simulink model "L1OF2_SecondOrder_M2_2_FRNEU"  (Simulink 7.8)
settings: Solver=ode45  StartTime=0.0  StopTime=10.0  FixedStep=1e-4
values from neighbouring files (symbols this model uses):
  a2 = M.den{1}(1)    [L1OF2SecondOrder2_2.m]
  Am = A_Db'    [L1OF2SecondOrder2_2.m]    (also in MaximiereL1NG.m)
  bm = c_Db'    [L1OF2SecondOrder2_2.m]    (also in MaximiereL1NG.m)
  cm = b_Db'    [L1OF2SecondOrder2_2.m]    (also in MaximiereL1NG.m)
  epsilon = 1.3    [L1OF2SecondOrder2_2.m]
  Gain = -Phi\mu1    [L1OF2SecondOrder2_2.m]
  ICy = 0    [L1OF2SecondOrder2_2.m]
  KmY = 2.4    [L1OF2SecondOrder2_2.m]
  kvy = 0    [L1OF2SecondOrder2_2.m]
  m = 19    [L1OF2SecondOrder2_2.m]
  M = 1/(7.713778844*s^2+10.06175892*s+1)    [L1OF2SecondOrder2_2.m]    (also in MaximiereL1NG.m = 1/(1.566434557*s^2+3.001699185*s+1))
  pD = p(2)-a1/a2    [L1OF2SecondOrder2_2.m]
  pI = p(4)    [L1OF2SecondOrder2_2.m]
  pK = p(3)-a0/a2    [L1OF2SecondOrder2_2.m]
  Ref_Amplitude = 0.3/Ref_Frequenz^2    (= 0.0697804295057)    [L1OF2SecondOrder2_2.m]
  Ref_Frequenz = 2*pi*0.33    (= 2.07345115137)    [L1OF2SecondOrder2_2.m]
  ST = 0.0005    [L1OF2SecondOrder2_2.m]
  Tt = 0.0667    [L1OF2SecondOrder2_2.m]
undefined symbols (not defined in the file or in its folder): d1, d2, delta, FpxLookUp1, FpxLookUp2, FpyLookUp1, FpyLookUp2, ICphi, ICvphi, ICvx, ICvy, ICx, J, KmX, kvphi, kvx, KX1, KX2, KY1, KY2, Ox1, Ox2, Oy1, Oy2, phx, phy, sigma, Tk, Vx1, Vx2, Vy1, Vy2, xLookUp1, xLookUp2, yLookUp1, yLookUp2
libraries: cstblocks x3, simulink x3
settings Model: Creator=Markus  LastModifiedBy=Markus

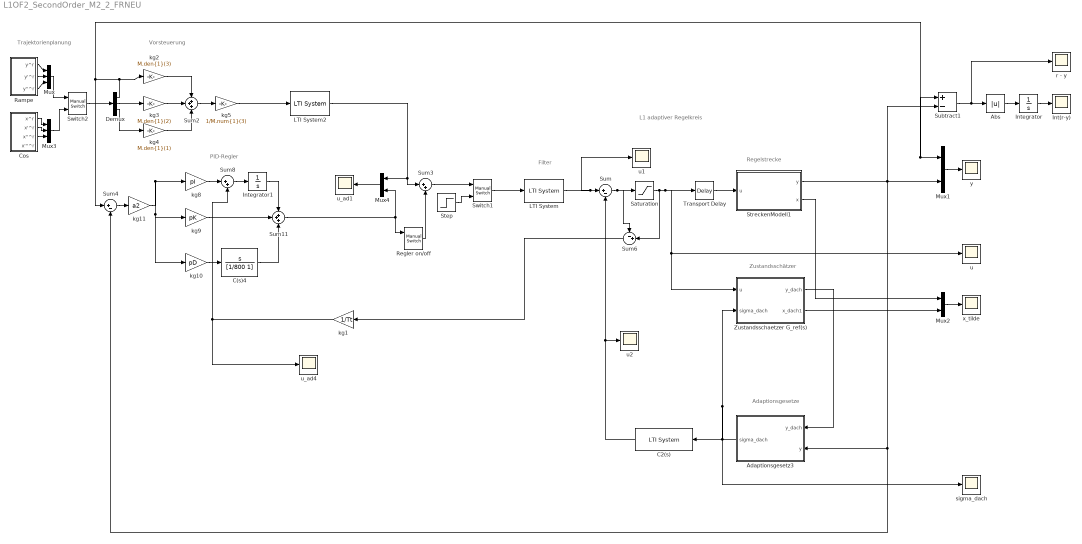
== system L1OF2_SecondOrder_M2_2_FRNEU ==
  note: Filter
  note: Zustandsschätzer
  note: Adaptionsgesetze
  note: Regelstrecke
  note: Trajektorienplanung
  note: Vorsteuerung
  note: L1 adaptiver Regelkreis
  note: PID-Regler
  Abs : Abs
  Adaptionsgesetz3 : Subsystem
  C(s)4 : TransferFcn  Numerator=[1 0]  Denominator=[1/800 1]
  C2(s) : cstblocks/LTI System  sys=C2  IC=[]
  Cos : Subsystem
  Demux : Demux  Outputs=3
  Int(r-y) : Scope
      settings: TimeRange=6  YMin=0.18335  YMax=0.18445  SaveName=ScopeData2
  Integrator : Integrator
  Integrator1 : Integrator
  LTI System : cstblocks/LTI System  sys=C  IC=[]
  LTI System2 : cstblocks/LTI System  sys=C_inv  IC=[]
  Mux : Mux  Inputs=3
  Mux1 : Mux  Inputs=2
  Mux2 : Mux  Inputs=2
  Mux3 : Mux  Inputs=3
  Mux4 : Mux  Inputs=3
  Rampe : Subsystem
  Regler on/off : simulink/Signal Routing/Manual Switch  sw=1  action=0  varsize=off
  Saturation : Saturate  UpperLimit=3  LowerLimit=-3
  Step : Step  After=0.06  SampleTime=0
  StreckenModell1 : Subsystem
  Subtract1 : Sum  Inputs=+-
  Sum : Sum  Inputs=|+-
  Sum11 : Sum  Inputs=+++
  Sum2 : Sum  Inputs=+++
  Sum3 : Sum  Inputs=|++
  Sum4 : Sum  Inputs=|+-
  Sum6 : Sum  Inputs=-+|
  Sum8 : Sum  Inputs=|++
  Switch1 : simulink/Signal Routing/Manual Switch  sw=1  action=0  varsize=off
  Switch2 : simulink/Signal Routing/Manual Switch  sw=1  action=0  varsize=off
  Transport Delay : TransportDelay  DelayTime=0.000
  Zustandsschaetzer G_ref(s) : Subsystem
  kg1 : Gain  Gain=1/Tt
  kg10 : Gain  Gain=pD
  kg11 : Gain  Gain=a2
  kg2 : Gain  Gain=M.den{1}(3)
  kg3 : Gain  Gain=M.den{1}(2)
  kg4 : Gain  Gain=M.den{1}(1)
  kg5 : Gain  Gain=1/M.num{1}(3)
  kg8 : Gain  Gain=pI
  kg9 : Gain  Gain=pK
  r - y : Scope
      settings: TimeRange=10  YMin=6e-012  YMax=2.6e-011  SaveName=simoutE
  sigma_dach : Scope
      settings: TimeRange=10  YMin=-0.04  YMax=0.075  SaveName=simoutS
  u : Scope
      settings: TimeRange=8  YMin=-2  YMax=2  SaveName=simoutU
  u1 : Scope
      settings: TimeRange=10  YMin=0.37  YMax=0.56  SaveName=ScopeData13
  u2 : Scope
      settings: TimeRange=10  YMin=-17.5  YMax=37.5  SaveName=ScopeData12
  u_ad1 : Scope
      settings: TimeRange=20  YMin=-50  YMax=110  SaveName=simoutV
  u_ad4 : Scope
      settings: TimeRange=20  YMin=-170  YMax=50  SaveName=simoutV1
  x_tilde : Scope
      settings: TimeRange=10  YMin=-0.0075  YMax=0.0475  SaveName=simoutU1
  y : Scope
      settings: TimeRange=4  YMin=0.07778  YMax=0.07781  SaveName=simout
  wires:
  Mux1/1 -> y/1
  Adaptionsgesetz3/1(sigma_dach) -> Zustandsschaetzer G_ref(s)/2(sigma_dach), sigma_dach/1, C2(s)/1
  Zustandsschaetzer G_ref(s)/1(y_dach) -> Adaptionsgesetz3/1(y_dach)
  LTI System/1 -> Sum/1, u1/1
  C2(s)/1 -> Sum/2, u2/1
  Subtract1/1 -> r - y/1, Abs/1
  Integrator/1 -> Int(r-y)/1
  Abs/1 -> Integrator/1
  Sum/1 -> Saturation/1, Sum6/1
  Saturation/1 -> Zustandsschaetzer G_ref(s)/1(u), u/1, Transport Delay/1, Sum6/2
  Switch1/1 -> LTI System/1
  StreckenModell1/1(y) -> Mux1/2, Adaptionsgesetz3/2(y), Sum4/2, Subtract1/2
  Transport Delay/1 -> StreckenModell1/1(u)
  Mux2/1 -> x_tilde/1
  StreckenModell1/2(x) -> Mux2/1
  Zustandsschaetzer G_ref(s)/2(x_dach1) -> Mux2/2
  Demux/1 -> kg2/1, Sum4/1, Subtract1/1, Mux1/1
  Demux/2 -> kg3/1
  Demux/3 -> kg4/1
  kg3/1 -> Sum2/2
  kg4/1 -> Sum2/3
  Sum2/1 -> kg5/1
  kg2/1 -> Sum2/1
  Rampe/1(y^r) -> Mux/1
  Rampe/2(y'^r) -> Mux/2
  Rampe/3(y''^r) -> Mux/3
  Mux/1 -> Switch2/1
  Switch2/1 -> Demux/1
  Mux3/1 -> Switch2/2
  Cos/1(x^r) -> Mux3/1
  Cos/2(x'^r) -> Mux3/2
  Cos/3(x''^r) -> Mux3/3
  Mux4/1 -> u_ad1/1
  Regler on/off/1 -> Sum3/2
  Sum3/1 -> Switch1/1
  kg5/1 -> LTI System2/1
  LTI System2/1 -> Sum3/1, Mux4/1
  kg1/1 -> Sum8/2, u_ad4/1
  Integrator1/1 -> Sum11/1
  kg9/1 -> Sum11/2
  kg8/1 -> Sum8/1
  Sum8/1 -> Integrator1/1
  kg10/1 -> C(s)4/1
  C(s)4/1 -> Sum11/3
  kg11/1 -> kg8/1, kg9/1, kg10/1
  Step/1 -> Switch1/2
  Sum4/1 -> kg11/1
  Sum11/1 -> Regler on/off/1, Mux4/3
  Sum6/1 -> kg1/1

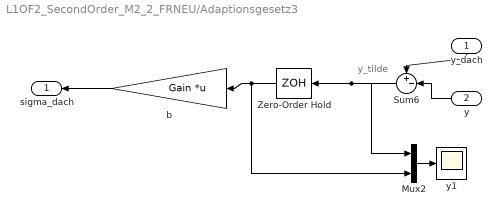
== system L1OF2_SecondOrder_M2_2_FRNEU/Adaptionsgesetz3 ==
  note: y_tilde
  y_dach : Inport
  y : Inport  Port=2
  Mux2 : Mux  Inputs=2
  Sum6 : Sum  Inputs=+-|
  Zero-Order Hold : ZeroOrderHold  SampleTime=ST
  b : Gain  Gain=Gain  Multiplication=Matrix(K*u)
  y1 : Scope
      settings: TimeRange=10  YMin=-0.004500000000000001  YMax=0  SaveName=ScopeData4
  sigma_dach : Outport
  wires:
  Sum6/1 -> Zero-Order Hold/1, Mux2/1
  y_dach/1 -> Sum6/1
  y/1 -> Sum6/2
  Zero-Order Hold/1 -> b/1, Mux2/2
  b/1 -> sigma_dach/1
  Mux2/1 -> y1/1

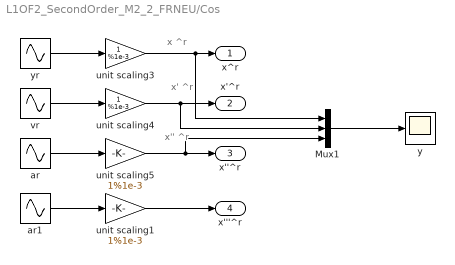
== system L1OF2_SecondOrder_M2_2_FRNEU/Cos ==
  note: x ^r
  note: x' ^r
  note: x'' ^r
  Mux1 : Mux  Inputs=3
  ar : Sin  Amplitude=-Ref_Amplitude*Ref_Frequenz^2  Frequency=Ref_Frequenz  Phase=pi/2  SampleTime=0
  ar1 : Sin  Amplitude=Ref_Amplitude*Ref_Frequenz^3  Frequency=Ref_Frequenz  SampleTime=0
  unit scaling1 : Gain  Gain=1%1e-3
  unit scaling3 : Gain  Gain=1 %1e-3
  unit scaling4 : Gain  Gain=1 %1e-3
  unit scaling5 : Gain  Gain=1%1e-3
  vr : Sin  Amplitude=-Ref_Amplitude*Ref_Frequenz  Frequency=Ref_Frequenz  SampleTime=0
  y : Scope
      settings: TimeRange=20  YMin=-0.3  YMax=0.25  SaveName=simout1
  yr : Sin  Amplitude=Ref_Amplitude  Frequency=Ref_Frequenz  Phase=pi/2  SampleTime=0
  x^r : Outport
  x'^r : Outport  Port=2
  x''^r : Outport  Port=3
  x'''^r : Outport  Port=4
  wires:
  ar/1 -> unit scaling5/1
  vr/1 -> unit scaling4/1
  yr/1 -> unit scaling3/1
  unit scaling3/1 -> x^r/1, Mux1/1
  unit scaling4/1 -> x'^r/1, Mux1/2
  unit scaling5/1 -> x''^r/1, Mux1/3
  Mux1/1 -> y/1
  ar1/1 -> unit scaling1/1
  unit scaling1/1 -> x'''^r/1

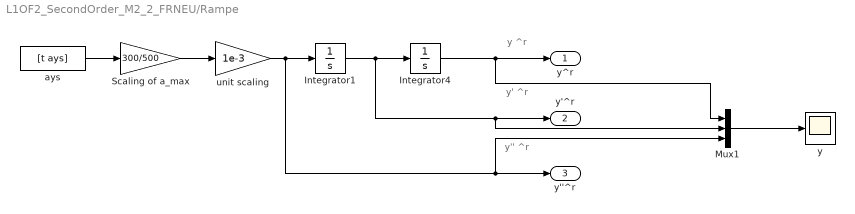
== system L1OF2_SecondOrder_M2_2_FRNEU/Rampe ==
  note: y ^r
  note: y' ^r
  note: y'' ^r
  Integrator1 : Integrator  InitialCondition=ICvy
  Integrator4 : Integrator  InitialCondition=ICy
  Mux1 : Mux  Inputs=3
  Scaling of a_max : Gain  Gain=300/500
  ays : FromWorkspace  VariableName=[t ays]  SampleTime=0
  unit scaling : Gain  Gain=1e-3
  y : Scope
      settings: TimeRange=20  YMin=-0.005  YMax=0.08  SaveName=simout2
  y^r : Outport
  y'^r : Outport  Port=2
  y''^r : Outport  Port=3
  wires:
  ays/1 -> Scaling of a_max/1
  Scaling of a_max/1 -> unit scaling/1
  Integrator1/1 -> Integrator4/1, y'^r/1, Mux1/2
  unit scaling/1 -> Integrator1/1, y''^r/1, Mux1/3
  Integrator4/1 -> y^r/1, Mux1/1
  Mux1/1 -> y/1

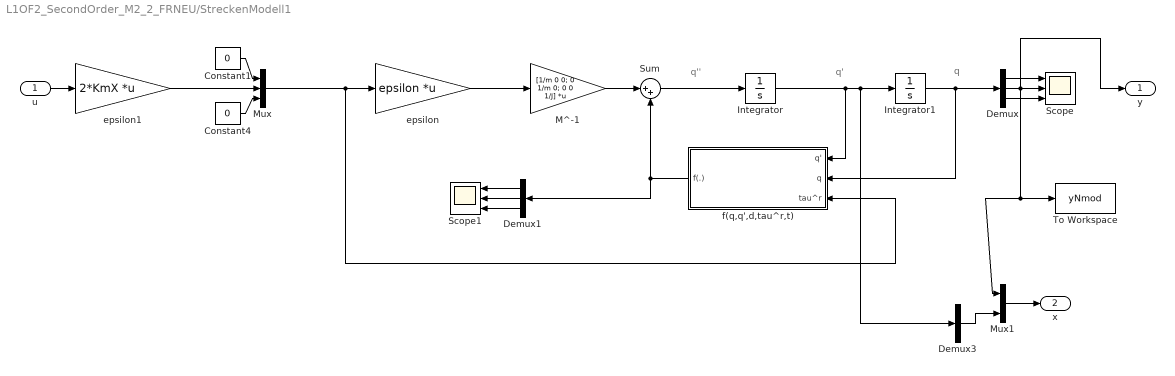
== system L1OF2_SecondOrder_M2_2_FRNEU/StreckenModell1 ==
  note: q
  note: q'
  note: q''
  u : Inport
  Constant1 : Constant  Value=0
  Constant4 : Constant  Value=0
  Demux : Demux  Outputs=3
  Demux1 : Demux  Outputs=3
  Demux3 : Demux  Outputs=3
  Integrator : Integrator  InitialCondition=[ICvx;ICvy;ICvphi]
  Integrator1 : Integrator  InitialCondition=[ICx;ICy;ICphi]
  M^-1 : Gain  Gain=[1/m 0 0; 0 1/m 0; 0 0 1/J]  Multiplication=Matrix(K*u)
  Mux : Mux  Inputs=3
  Mux1 : Mux  Inputs=2
  Scope : Scope  NumInputPorts=3
      settings: YMin=0.0014~0.0425~-1.73472e-018  YMax=0.0029~0.0625~0.08
  Scope1 : Scope  NumInputPorts=3
      settings: YMin=-1~1.1~-1  YMax=1~2.6~1  SaveName=ScopeData2
  Sum : Sum  Inputs=|++
  To Workspace : ToWorkspace  VariableName=yNmod  SampleTime=-1  SaveFormat=Structure With Time
  epsilon : Gain  Gain=epsilon  Multiplication=Matrix(K*u)
  epsilon1 : Gain  Gain=2*KmX  Multiplication=Matrix(K*u)
  f(q,q',d,tau^r,t) : Subsystem
  y : Outport
  x : Outport  Port=2
  wires:
  Demux3/2 -> Mux1/2
  Mux1/1 -> x/1
  Constant4/1 -> Mux/3
  Constant1/1 -> Mux/1
  Mux/1 -> f(q,q',d,tau^r,t)/3(tau^r), epsilon/1
  Demux1/3 -> Scope1/3
  Demux1/2 -> Scope1/2
  Demux1/1 -> Scope1/1
  f(q,q',d,tau^r,t)/1(f(.)) -> Demux1/1, Sum/2
  epsilon/1 -> M^-1/1
  Integrator1/1 -> f(q,q',d,tau^r,t)/2(q), Demux/1
  Sum/1 -> Integrator/1
  M^-1/1 -> Sum/1
  Integrator/1 -> Demux3/1, Integrator1/1, f(q,q',d,tau^r,t)/1(q')
  Demux/3 -> Scope/3
  Demux/2 -> Mux1/1, To Workspace/1, y/1, Scope/2
  Demux/1 -> Scope/1
  u/1 -> epsilon1/1
  epsilon1/1 -> Mux/2

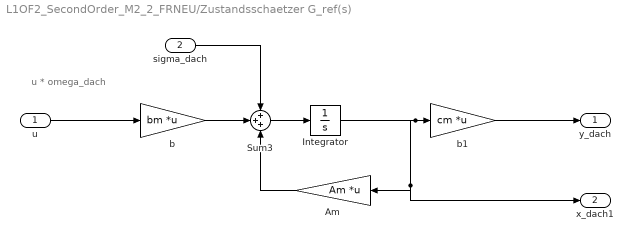
== system L1OF2_SecondOrder_M2_2_FRNEU/Zustandsschaetzer G_ref(s) ==
  note: u * omega_dach
  u : Inport
  sigma_dach : Inport  Port=2
  Am : Gain  Gain=Am  Multiplication=Matrix(K*u)
  Integrator : Integrator
  Sum3 : Sum  Inputs=+++
  b : Gain  Gain=bm  Multiplication=Matrix(K*u)
  b1 : Gain  Gain=cm  Multiplication=Matrix(K*u)
  y_dach : Outport
  x_dach1 : Outport  Port=2
  wires:
  Integrator/1 -> b1/1, Am/1, x_dach1/1
  Sum3/1 -> Integrator/1
  Am/1 -> Sum3/3
  b/1 -> Sum3/2
  sigma_dach/1 -> Sum3/1
  b1/1 -> y_dach/1
  u/1 -> b/1

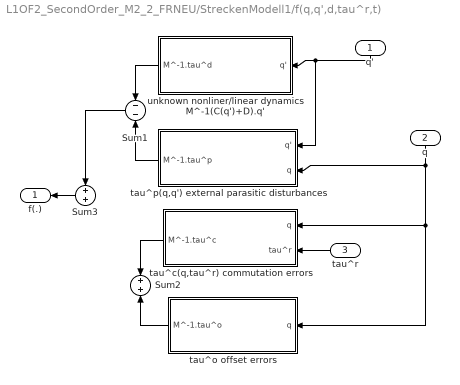
== system L1OF2_SecondOrder_M2_2_FRNEU/StreckenModell1/f(q,q',d,tau^r,t) ==
  q' : Inport
  q : Inport  Port=2
  tau^r : Inport  Port=3
  Sum1 : Sum  Inputs=--
  Sum2 : Sum
  Sum3 : Sum
  tau^c(q,tau^r) commutation errors : Subsystem
  tau^o offset errors : Subsystem
  tau^p(q,q') external parasitic disturbances : Subsystem
  unknown nonliner/linear dynamics M^-1(C(q')+D).q' : Subsystem
  f(.) : Outport
  wires:
  Sum3/1 -> f(.)/1
  tau^r/1 -> tau^c(q,tau^r) commutation errors/2(tau^r)
  q/1 -> tau^o offset errors/1(q), tau^c(q,tau^r) commutation errors/1(q), tau^p(q,q') external parasitic disturbances/2(q)
  q'/1 -> unknown nonliner/linear dynamics M^-1(C(q')+D).q'/1(q'), tau^p(q,q') external parasitic disturbances/1(q')
  Sum1/1 -> Sum3/1
  unknown nonliner/linear dynamics M^-1(C(q')+D).q'/1(M^-1.tau^d) -> Sum1/1
  tau^c(q,tau^r) commutation errors/1(M^-1.tau^c) -> Sum2/1
  tau^p(q,q') external parasitic disturbances/1(M^-1.tau^p) -> Sum1/2
  tau^o offset errors/1(M^-1.tau^o) -> Sum2/2

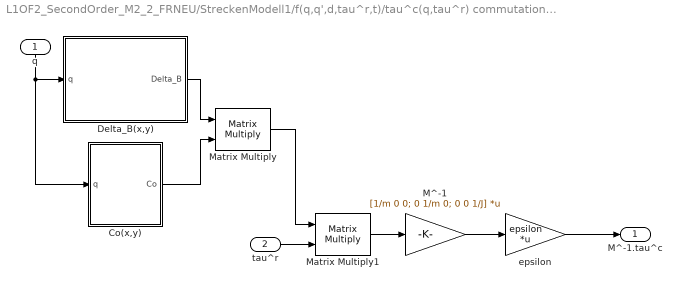
== system L1OF2_SecondOrder_M2_2_FRNEU/StreckenModell1/f(q,q',d,tau^r,t)/tau^c(q,tau^r) commutation errors ==
  q : Inport
  tau^r : Inport  Port=2
  Co(x,y) : MATLAB Function  TreatAsAtomicUnit=on
  Delta_B(x,y) : MATLAB Function  TreatAsAtomicUnit=on
  "M^-1  " : Gain  Gain=[1/m 0 0; 0 1/m 0; 0 0 1/J]  Multiplication=Matrix(K*u)
  Matrix Multiply : Product  Multiplication=Matrix(*)
  Matrix Multiply1 : Product  Multiplication=Matrix(*)
  epsilon : Gain  Gain=epsilon  Multiplication=Matrix(K*u)
  M^-1.tau^c : Outport
  wires:
  "M^-1  "/1 -> epsilon/1
  epsilon/1 -> M^-1.tau^c/1
  tau^r/1 -> Matrix Multiply1/2
  q/1 -> Co(x,y)/1(q), Delta_B(x,y)/1(q)
  Matrix Multiply1/1 -> "M^-1  "/1
  Matrix Multiply/1 -> Matrix Multiply1/1
  Co(x,y)/1(Co) -> Matrix Multiply/2
  Delta_B(x,y)/1(Delta_B) -> Matrix Multiply/1

== system L1OF2_SecondOrder_M2_2_FRNEU/StreckenModell1/f(q,q',d,tau^r,t)/tau^o offset errors ==
  q : Inport
  Delta_B(x,y) : MATLAB Function  TreatAsAtomicUnit=on
  "M^-1  " : Gain  Gain=[1/m 0 0; 0 1/m 0; 0 0 1/J]  Multiplication=Matrix(K*u)
  Matrix Multiply1 : Product  Multiplication=Matrix(*)
  sigma : Constant  Value=sigma
  M^-1.tau^o : Outport
  wires:
  sigma/1 -> Matrix Multiply1/2
  Matrix Multiply1/1 -> "M^-1  "/1
  "M^-1  "/1 -> M^-1.tau^o/1
  q/1 -> Delta_B(x,y)/1(q)
  Delta_B(x,y)/1(Bp) -> Matrix Multiply1/1

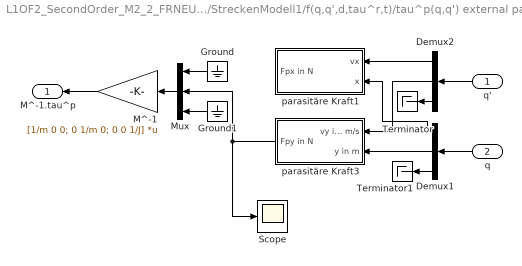
== system L1OF2_SecondOrder_M2_2_FRNEU/StreckenModell1/f(q,q',d,tau^r,t)/tau^p(q,q') external parasitic disturbances ==
  q' : Inport
  q : Inport  Port=2
  Demux1 : Demux  Outputs=3
  Demux2 : Demux  Outputs=3
  Ground : Ground
  Ground1 : Ground
  "M^-1  " : Gain  Gain=[1/m 0 0; 0 1/m 0; 0 0 1/J]  Multiplication=Matrix(K*u)
  Mux : Mux  Inputs=3
  Scope : Scope
      settings: YMin=-4.06576e-020  YMax=0.0007  SaveName=ScopeData19
  Terminator : Terminator
  Terminator1 : Terminator
  parasitäre Kraft1 : Subsystem
  parasitäre Kraft3 : Subsystem
  M^-1.tau^p : Outport
  wires:
  Ground1/1 -> Mux/3
  "M^-1  "/1 -> M^-1.tau^p/1
  Mux/1 -> "M^-1  "/1
  q/1 -> Demux1/1
  q'/1 -> Demux2/1
  parasitäre Kraft3/1(Fpy in N) -> Scope/1, Mux/2
  Demux2/2 -> parasitäre Kraft3/1(vy in m/s)
  Demux1/3 -> Terminator1/1
  Demux2/3 -> Terminator/1
  Demux2/1 -> parasitäre Kraft1/1(vx)
  Demux1/2 -> parasitäre Kraft3/2(y in m)
  Demux1/1 -> parasitäre Kraft1/2(x)
  Ground/1 -> Mux/1

== system L1OF2_SecondOrder_M2_2_FRNEU/StreckenModell1/f(q,q',d,tau^r,t)/unknown nonliner/linear dynamics M^-1(C(q')+D).q' ==
  q' : Inport
  C(q').q' : Subsystem
  "M^-1 " : Gain  Gain=[1/m 0 0; 0 1/m 0; 0 0 1/J]  Multiplication=Matrix(K*u)
  M^-1.D : Gain  Gain=[kvx/m 0 0; 0 kvy/m 0; 0 0 kvphi/J]  Multiplication=Matrix(K*u)
  Sum1 : Sum
  M^-1.tau^d : Outport
  wires:
  M^-1.D/1 -> Sum1/1
  Sum1/1 -> M^-1.tau^d/1
  "M^-1 "/1 -> Sum1/2
  q'/1 -> C(q').q'/1(q'), M^-1.D/1
  C(q').q'/1(C(q').q') -> "M^-1 "/1

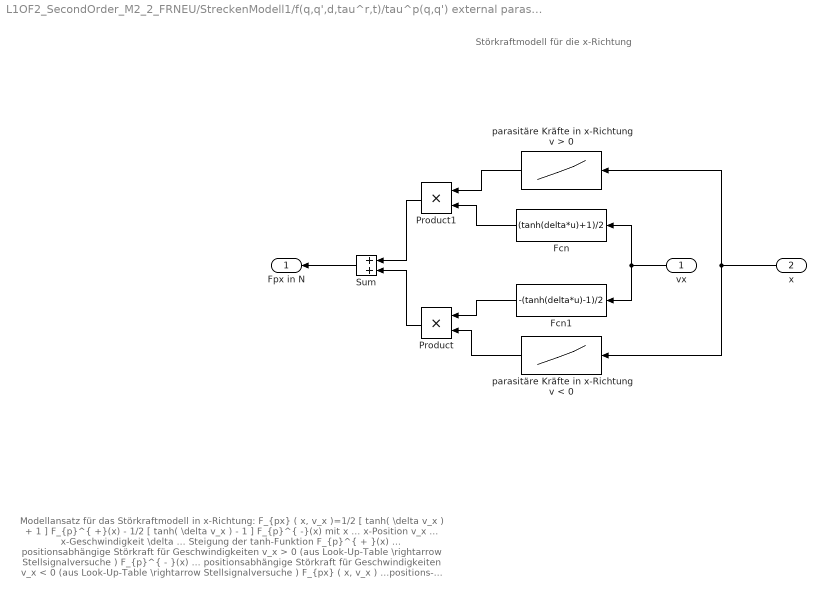
== system L1OF2_SecondOrder_M2_2_FRNEU/StreckenModell1/f(q,q',d,tau^r,t)/tau^p(q,q') external parasitic disturbances/parasitäre Kraft1 ==
  note: Modellansatz für das Störkraftmodell in x-Richtung:
      |
      | F_{px} ( x, v_x )=1/2 [ tanh(  \delta  v_x ) + 1 ] F_{p}^{  +}(x)  -  1/2 [ tanh( \delta  v_x )  - 1 ]  F_{p}^{  -}(x)
      |
      | mit
      |
      | x    ... x-Position
      | v_x  ... x-Geschwindigkeit
      | \delta   ... Steigung der tanh-Funktion
      |
      | F_{p}^{  + }(x)          ... positionsabhängige Störkraft für Geschwindigkeiten v_x   >  0  (aus Look-Up-Table \rightarrow Stellsignalversuche )
      | F_{p}^{  - }(x)           ... positionsabhängige Störkraft für Geschwindigkeiten v_x   <  0  (aus Look-Up-Table \rightarrow Stellsignalversuche )
      | F_{px} ( x, v_x ) ...positions- und richtungsabhängige Störkraft
  note: Störkraftmodell für die x-Richtung
  vx : Inport
  x : Inport  Port=2
  Fcn : Fcn  Expr=(tanh(delta*u)+1)/2
  Fcn1 : Fcn  Expr=-(tanh(delta*u)-1)/2
  Product : Product  RndMeth=Zero
  Product1 : Product  RndMeth=Zero
  Sum : Sum
  parasitäre Kräfte in x-Richtung v < 0 : Lookup_n-D  NumberOfTableDimensions=1  BreakpointsForDimension1=fliplr(xLookUp2')*1e-3+Vx2  Table=fliplr(FpxLookUp2')*KX2+Ox2  InterpMethod=Cubic spline  RndMeth=Simplest  InputSameDT=on
  parasitäre Kräfte in x-Richtung v > 0 : Lookup_n-D  NumberOfTableDimensions=1  BreakpointsForDimension1=xLookUp1*1e-3+Vx1  Table=FpxLookUp1*KX1+Ox1  InterpMethod=Cubic spline  RndMeth=Simplest  InputSameDT=on
  Fpx in N : Outport
  wires:
  vx/1 -> Fcn1/1, Fcn/1
  Sum/1 -> Fpx in N/1
  Product/1 -> Sum/2
  Product1/1 -> Sum/1
  Fcn/1 -> Product1/2
  parasitäre Kräfte in x-Richtung v > 0/1 -> Product1/1
  Fcn1/1 -> Product/1
  parasitäre Kräfte in x-Richtung v < 0/1 -> Product/2
  x/1 -> parasitäre Kräfte in x-Richtung v < 0/1, parasitäre Kräfte in x-Richtung v > 0/1

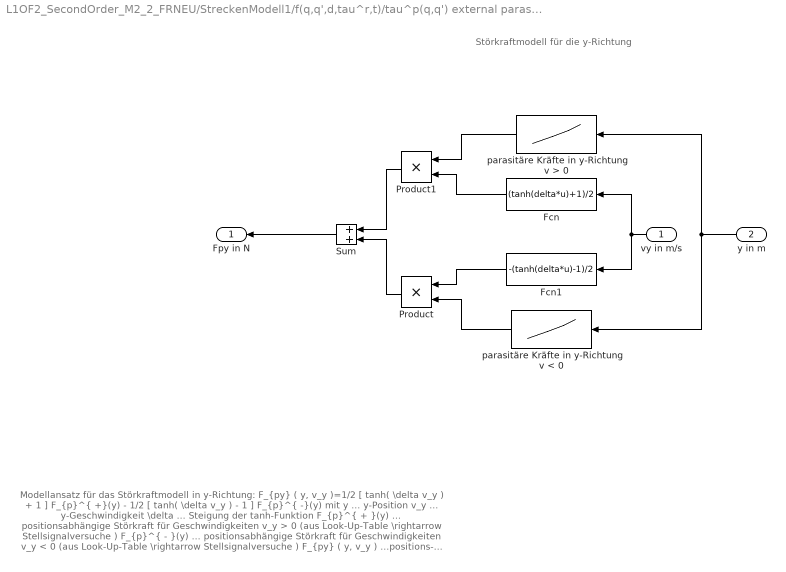
== system L1OF2_SecondOrder_M2_2_FRNEU/StreckenModell1/f(q,q',d,tau^r,t)/tau^p(q,q') external parasitic disturbances/parasitäre Kraft3 ==
  note: Störkraftmodell für die y-Richtung
  note: Modellansatz für das Störkraftmodell in y-Richtung:
      |
      | F_{py} ( y, v_y )=1/2 [ tanh(  \delta  v_y ) + 1 ] F_{p}^{  +}(y)  -  1/2 [ tanh( \delta  v_y )  - 1 ]  F_{p}^{  -}(y)
      |
      | mit
      |
      | y    ... y-Position
      | v_y  ... y-Geschwindigkeit
      | \delta   ... Steigung der tanh-Funktion
      |
      | F_{p}^{  + }(y)          ... positionsabhängige Störkraft für Geschwindigkeiten v_y   >  0  (aus Look-Up-Table \rightarrow Stellsignalversuche )
      | F_{p}^{  - }(y)           ... positionsabhängige Störkraft für Geschwindigkeiten v_y   <  0  (aus Look-Up-Table \rightarrow Stellsignalversuche )
      | F_{py} ( y, v_y ) ...positions- und richtungsabhängige Störkraft
  vy in m/s : Inport
  y in m : Inport  Port=2
  Fcn : Fcn  Expr=(tanh(delta*u)+1)/2
  Fcn1 : Fcn  Expr=-(tanh(delta*u)-1)/2
  Product : Product  RndMeth=Zero
  Product1 : Product  RndMeth=Zero
  Sum : Sum
  parasitäre Kräfte in y-Richtung v < 0 : Lookup_n-D  NumberOfTableDimensions=1  BreakpointsForDimension1=fliplr(yLookUp2')*1e-3+Vy2  Table=fliplr(FpyLookUp2')*KY2+Oy2  InterpMethod=Cubic spline  RndMeth=Simplest  InputSameDT=on
  parasitäre Kräfte in y-Richtung v > 0 : Lookup_n-D  NumberOfTableDimensions=1  BreakpointsForDimension1=yLookUp1*1e-3+Vy1  Table=FpyLookUp1*KY1+Oy1  InterpMethod=Cubic spline  RndMeth=Simplest  InputSameDT=on
  Fpy in N : Outport
  wires:
  parasitäre Kräfte in y-Richtung v < 0/1 -> Product/2
  parasitäre Kräfte in y-Richtung v > 0/1 -> Product1/1
  Product/1 -> Sum/2
  Product1/1 -> Sum/1
  Fcn/1 -> Product1/2
  Fcn1/1 -> Product/1
  Sum/1 -> Fpy in N/1
  vy in m/s/1 -> Fcn/1, Fcn1/1
  y in m/1 -> parasitäre Kräfte in y-Richtung v > 0/1, parasitäre Kräfte in y-Richtung v < 0/1

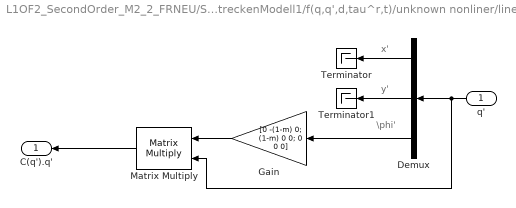
== system L1OF2_SecondOrder_M2_2_FRNEU/StreckenModell1/f(q,q',d,tau^r,t)/unknown nonliner/linear dynamics M^-1(C(q')+D).q'/C(q').q' ==
  note: \phi'
  note: y'
  note: x'
  q' : Inport
  Demux : Demux  Outputs=3
  Gain : Gain  Gain=[0 -(1-m) 0; (1-m) 0 0; 0 0 0]
  Matrix Multiply : Product  Multiplication=Matrix(*)
  Terminator : Terminator
  Terminator1 : Terminator
  C(q').q' : Outport
  wires:
  Demux/3 -> Gain/1
  Matrix Multiply/1 -> C(q').q'/1
  Gain/1 -> Matrix Multiply/1
  Demux/2 -> Terminator1/1
  Demux/1 -> Terminator/1
  q'/1 -> Matrix Multiply/2, Demux/1

== matlab function StreckenModell1/f(q,q',d,tau^r,t)/tau^c(q,tau^r) commutation errors/Co(x,y) ==
  data: q input double; Co output double; Tk parameter double; KmX parameter double; KmY parameter double; phx parameter double; phy parameter double; d1 parameter double; d2 parameter double
function Co = compute_Co(q,Tk,KmX,KmY,phx,phy,d1,d2)
%#codegen
x=q(1);
y=q(2);

% Flussdichte entlang der x- und y-Richtungen
B1x=sin(2*pi/Tk*x+phx+pi/2); %+
B2x=cos(2*pi/Tk*x+phx-pi/2); %-
B1y=sin(2*pi/Tk*y+phy);
B2y=cos(2*pi/Tk*y+phy);


Co =[B1x/(2*KmX)    0         d1*KmX*B1x/(2*(d1^2*KmX^2+d2^2*KmY^2));
     B2x/(2*KmX)    0         d1*KmX*B2x/(2*(d1^2*KmX^2+d2^2*KmY^2));
     B1x/(2*KmX)    0        -d1*KmX*B1x/(2*(d1^2*KmX^2+d2^2*KmY^2));
     B2x/(2*KmX)    0        -d1*KmX*B2x/(2*(d1^2*KmX^2+d2^2*KmY^2));
        0        B1y/(2*KmY) -d2*KmY*B1y/(2*(d1^2*KmX^2+d2^2*KmY^2));
        0        B2y/(2*KmY) -d2*KmY*B2y/(2*(d1^2*KmX^2+d2^2*KmY^2));
        0        B1y/(2*KmY)  d2*KmY*B1y/(2*(d1^2*KmX^2+d2^2*KmY^2));
        0        B2y/(2*KmY)  d2*KmY*B2y/(2*(d1^2*KmX^2+d2^2*KmY^2))];

== matlab function StreckenModell1/f(q,q',d,tau^r,t)/tau^c(q,tau^r) commutation errors/Delta_B(x,y) ==
  data: q input double; Delta_B output double; Tk parameter double; KmX parameter double; KmY parameter double; phx parameter double; phy parameter double; d1 parameter double; d2 parameter double
function Delta_B = compute_Delta_B(q,Tk,KmX,KmY,phx,phy,d1,d2)
%#codegen
x=q(1);
y=q(2);

% Flussdichte entlang der x- und y-Richtungen
B1x=KmX*sin(2*pi/Tk*x+phx+pi/2); %+
B2x=KmX*cos(2*pi/Tk*x+phx-pi/2); %-
B1y=KmY*sin(2*pi/Tk*y+phy);
B2y=KmY*cos(2*pi/Tk*y+phy);

% nominelles Feld
B =[   B1x    B2x     B1x     B2x      0       0      0      0;
        0      0       0       0      B1y     B2y    B1y    B2y;
     d1*B1x d1*B2x -d1*B1x -d1*B2x -d2*B1y -d2*B2y d2*B1y d2*B2y];

 
% Fehlerhaftes Magnetfeld
maxBp=0.4704;
B1xp=0.4851*tanh(0.1877*sinh(3.104*B1x))/maxBp; 
B2xp=0.4851*tanh(0.1877*sinh(3.104*B2x))/maxBp; 
B1yp=0.4851*tanh(0.1877*sinh(3.104*B1y))/maxBp; 
B2yp=0.4851*tanh(0.1877*sinh(3.104*B2y))/maxBp; 

Bp =[   B1xp    B2xp    B1xp     B2xp      0       0       0       0;
         0       0       0        0       B1yp    B2yp    B1yp    B2yp;
     d1*B1xp d1*B2xp -d1*B1xp -d1*B2xp -d2*B1yp -d2*B2yp d2*B1yp d2*B2yp];
 
Delta_B=Bp-B;

== matlab function StreckenModell1/f(q,q',d,tau^r,t)/tau^o offset errors/Delta_B(x,y) ==
  data: q input double; Bp output double; Tk parameter double; KmX parameter double; KmY parameter double; phx parameter double; phy parameter double; d1 parameter double; d2 parameter double
function Bp = compute_Bp(q,Tk,KmX,KmY,phx,phy,d1,d2)
%#codegen
x=q(1);
y=q(2);

% Flussdichte entlang der x- und y-Richtungen
B1x=KmX*sin(2*pi/Tk*x+phx+pi/2); %+
B2x=KmX*cos(2*pi/Tk*x+phx-pi/2); %-
B1y=KmY*sin(2*pi/Tk*y+phy);
B2y=KmY*cos(2*pi/Tk*y+phy);
 
% Fehlerhaftes Magnetfeld
maxBp=0.4704;
B1xp=0.4851*tanh(0.1877*sinh(3.104*B1x))/maxBp; 
B2xp=0.4851*tanh(0.1877*sinh(3.104*B2x))/maxBp; 
B1yp=0.4851*tanh(0.1877*sinh(3.104*B1y))/maxBp; 
B2yp=0.4851*tanh(0.1877*sinh(3.104*B2y))/maxBp; 

Bp =[   B1xp    B2xp    B1xp     B2xp      0       0       0       0;
         0       0       0        0       B1yp    B2yp    B1yp    B2yp;
     d1*B1xp d1*B2xp -d1*B1xp -d1*B2xp -d2*B1yp -d2*B2yp d2*B1yp d2*B2yp];
